simulink model "Linear"  (R2016a)
settings: Solver=VariableStepAuto  StartTime=0.0  StopTime=10.0  RelTol=1e-3
undefined symbols (not defined in the file or in its folder): denumCo, numCo
libraries: simulink x1, vrlib x1
settings Model: Creator=asus  LastModifiedBy=asus

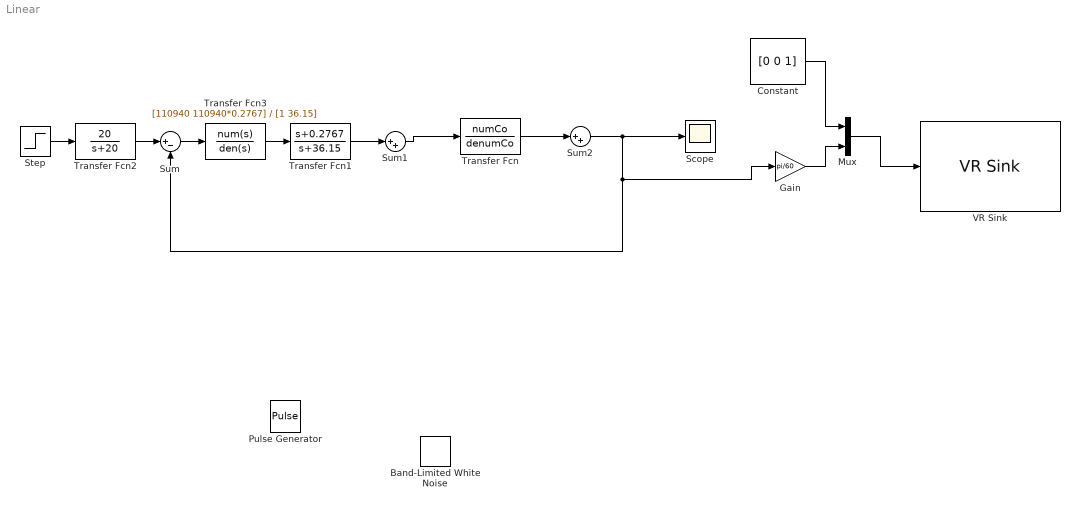
== system Linear ==
  Band-Limited White Noise : simulink/Sources/Band-Limited White Noise  Cov=[0.000001]  Ts=0.1  seed=[23341]
  Constant : Constant  Value=[0 0 1]
  Gain : Gain  Gain=pi/60
  Mux : Mux  Inputs=2
  Pulse Generator : DiscretePulseGenerator  PulseType=Time based  Amplitude=0.4  Period=5  PulseWidth=50
  Scope : Scope
  Step : Step  Time=0  SampleTime=0
  Sum : Sum  Inputs=|+-
  Sum1 : Sum  Inputs=|++
  Sum2 : Sum  Inputs=|++
  Transfer Fcn : TransferFcn  Numerator=numCo  Denominator=denumCo
  Transfer Fcn1 : TransferFcn  Numerator=[1 0.2767]  Denominator=[1 36.15]
  Transfer Fcn2 : TransferFcn  Numerator=[20]  Denominator=[1 20]
  Transfer Fcn3 : TransferFcn  Numerator=[110940 110940*0.2767]  Denominator=[1 36.15]
  VR Sink : vrlib/VR Sink  InstantiateOnLoad=on  SampleTime=0.1  ViewEnable=on  RemoteChange=off  RemoteView=off  FieldsWritten=joint.rotation.4.1.1.double  WorldFileName=talebi.WRL  AutoView=off  VideoDimensions=[]  AllowVariableSize=off
  wires:
  Sum/1 -> Transfer Fcn3/1
  Sum1/1 -> Transfer Fcn/1
  Transfer Fcn1/1 -> Sum1/1
  Transfer Fcn2/1 -> Sum/1
  Step/1 -> Transfer Fcn2/1
  Transfer Fcn/1 -> Sum2/1
  Sum2/1 -> Gain/1, Sum/2, Scope/1
  Transfer Fcn3/1 -> Transfer Fcn1/1
  Constant/1 -> Mux/1
  Gain/1 -> Mux/2
  Mux/1 -> VR Sink/1
